simulink model "mseDelay"  (R2023b)
settings: Solver=VariableStepAuto  StartTime=0.0  StopTime=10.0  RelTol=1e-3
settings Model: Creator=DarianMuresan  LastModifiedBy=DarianMuresan

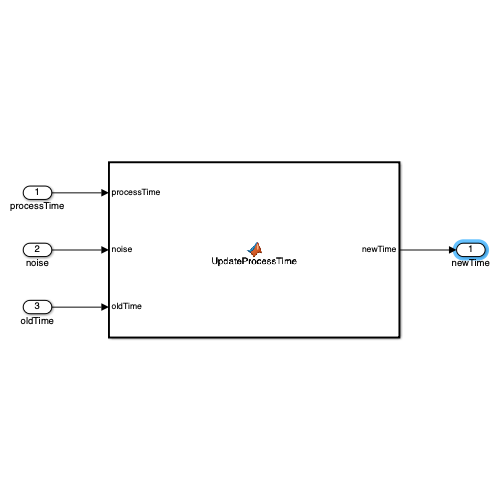
[thumbnail: Simulink's stored preview of the top-level diagram]
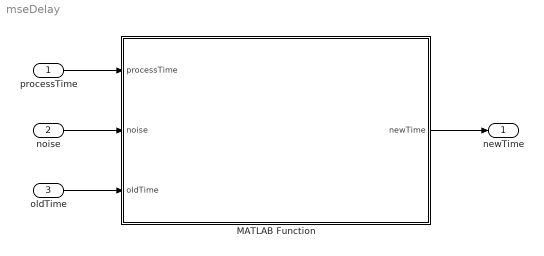
== system mseDelay ==
  processTime : Inport
  noise : Inport  Port=2
  oldTime : Inport  Port=3
  MATLAB Function : MATLAB Function  TreatAsAtomicUnit=on
  newTime : Outport
  wires:
  processTime/1 -> MATLAB Function/1(processTime)
  oldTime/1 -> MATLAB Function/3(oldTime)
  noise/1 -> MATLAB Function/2(noise)
  MATLAB Function/1(newTime) -> newTime/1

== matlab function mseDelay/MATLAB Function ==
  data: processTime input; newTime output; noise input; oldTime input
function newTime = mseDelay(processTime, noise, oldTime)

% Function to update the total time (add the delay) 
% based on the simple linear model of addition, 
% assuming the CPU times have already been calculated.
%
% Written by: Darian Muresan
% Modified last: October 10, 2024

if nargin<2
    noise = 0;
    oldTime = 0;
elseif nargin<3
    oldTime = 0;
end

if oldTime<0
    newTime = -1;
else
    % avoid negative time, since negative time implies path not taken
    newTime = max(oldTime+processTime+noise, 0);
end
